simulink model "subsys"  (R2018a)
settings: Solver=VariableStepAuto  StartTime=0.0  StopTime=30  RelTol=1e-3
values from neighbouring files (symbols this model uses):
  p = polyfit(x,d,7)    [matlab.m]
undefined symbols (not defined in the file or in its folder): J, magnitude
libraries: simulink x9, visionstatistics x1, neural x1, dspsrcs4 x1, dspxfrm3 x1, dspsigops x1
settings Model: Creator=Thinkpad  LastModifiedBy=Administrator

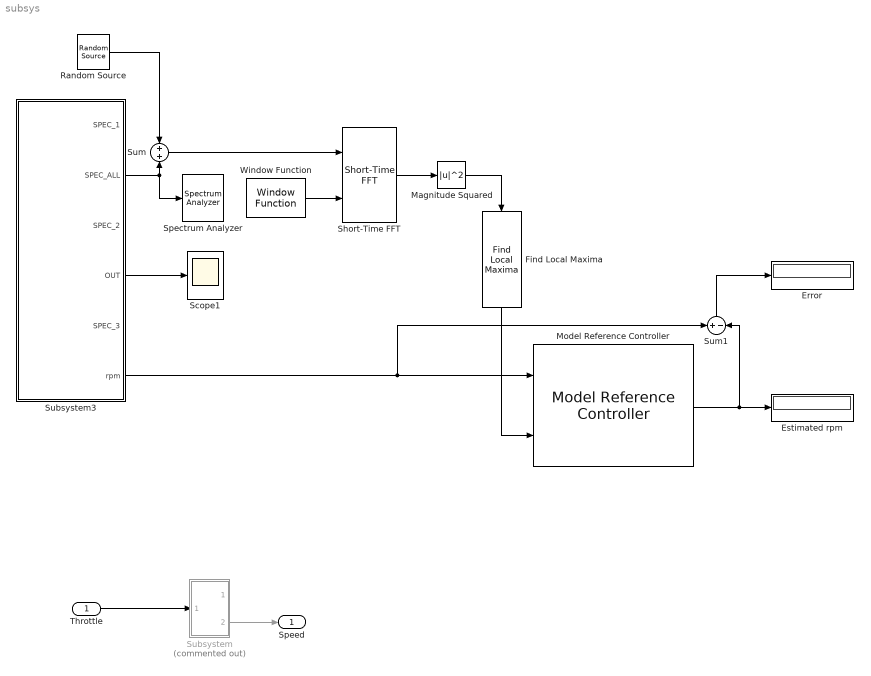
== system subsys ==
  Throttle : Inport
  Error : Display
  Estimated rpm : Display
  Find Local Maxima : visionstatistics/Find Local Maxima  num_peaks=2  nhood_size=[5 7]  src_thresh=Obsolete9b  src_thresh_inuse=Specify via dialog  threshold=10  inputIsHough=off  dt_peak=uint32  isOutVarDim=on  dt_count=uint32
      settings: SourceProductName=Computer Vision System Toolbox  SourceProductBaseCode=VP
  Magnitude Squared : Math  Operator=magnitude^2  SaturateOnIntegerOverflow=on
  Model Reference Controller : neural/Control Systems/Model Reference Controller  Nrc=[]  Nic=[]  Njc=[]  IW_y=[]  IW_u=[]  IW_r=[]  B1_c=[]  B2_c=[]  LW_c=[]  retraining_c=[]  max_i_int=[]  min_i_int=[]  max_r_int=[]  min_r_int=[]  Ts=[]  S1=[]  Ni=[]  Nj=[]  sim_file=0  trainfun=trainlm  Use_validation=[]  Use_Testing=[]  Use_Inc_training=[]  Use_previous_weights=[]  max_i=[]  min_i=[]  max_r=[]  min_r=[]  sam_training=[]  sam_training_c=[]  epochs=[]  epochs_c=[]  minp=[]  maxp=[]  mint=[]  maxt=[]  Normalize=[]  IW=[]  LW1_2=[]  LW2_1=[]  B1=[]  B2=[]  S1c=[]  Limit_output=[]  min_output=[]  max_output=[]  Ref_file=0
      settings: SourceProductName=Neural Network Toolbox  SourceProductBaseCode=NN
  Random Source : dspsrcs4/Random Source  SrcType=Gaussian  NormMethod=Ziggurat  CltLength=12  MinVal=0  MaxVal=1  MeanVal=0  VarVal=(0.05)^2  RepMode=Repeatable  rawSeed=1  IsInherit=off  SampMode=Discrete  SampTime=1/22050  SampFrame=512  DataType=Double  OutComplex=Real  OutputFrames=off
  Scope1 : Scope
  Short-Time FFT : dspxfrm3/Short-Time FFT  W=512  OvLap=384  M=1024
      settings: SourceProductName=DSP System Toolbox  SourceProductBaseCode=DS
  Spectrum Analyzer : SpectrumAnalyzer
  Subsystem : Subsystem  Commented=on
  Subsystem3 : Subsystem
  Sum : Sum
  Sum1 : Sum  Inputs=+-
  Window Function : dspsigops/Window Function  winmode=Generate window  wintype=Hamming  sampmode=Discrete  samptime=inf  N=512  Rs=50  beta=10  winsamp=Symmetric  UserWindow=hamming  OptParams=off  UserParams={'symmetric'}  dataType=double  isSigned=on  wordLen=16  udDataType=sfix(16)  fracBitsMode=Best precision  numFracBits=15  roundingMode=Floor  overflowMode=off  numSidelobes=4  sidelobeLevel=-30
      settings: SourceProductName=DSP System Toolbox  SourceProductBaseCode=DS
  Speed : Outport
  wires:
  Subsystem3/2(SPEC_ALL) -> Spectrum Analyzer/1, Sum/2
  Subsystem3/4(OUT) -> Scope1/1
  Window Function/1 -> Short-Time FFT/2
  Random Source/1 -> Sum/1
  Sum/1 -> Short-Time FFT/1
  Short-Time FFT/1 -> Magnitude Squared/1
  Magnitude Squared/1 -> Find Local Maxima/1
  Subsystem3/6(rpm) -> Sum1/1, Model Reference Controller/1
  Find Local Maxima/1 -> Model Reference Controller/2
  Model Reference Controller/1 -> Sum1/2, Estimated rpm/1
  Sum1/1 -> Error/1
  Throttle/1 -> Subsystem/1(Throttle)
  Subsystem/2(Speed) -> Speed/1

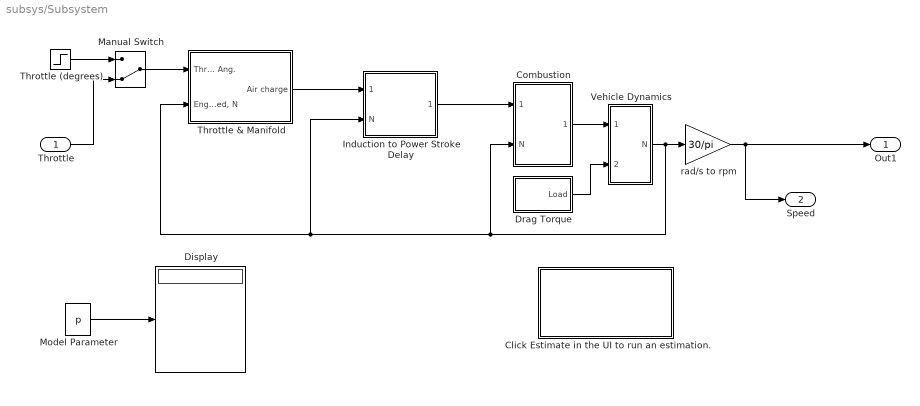
== system subsys/Subsystem ==
  Throttle : Inport
  Click Estimate in the UI to run an estimation. : Subsystem
      settings: OpenFcn=sdotool( slResolve('spe_speed_sdosession', 'spe_speed') );
      mask Display: disp('Parameter Estimation\nwith preloaded data')
  Combustion : Subsystem
  Display : Display
  Drag Torque : Subsystem
  Induction to Power Stroke Delay : Subsystem
  Manual Switch : ManualSwitch  CurrentSetting=0
  Model Parameter : Constant  Value=p
  Throttle (degrees) : Step  Time=2  Before=8.973  After=11  SampleTime=0
  Throttle & Manifold : Subsystem
  Vehicle Dynamics : Subsystem
  rad/s to rpm : Gain  Gain=30/pi  SaturateOnIntegerOverflow=on  OutDataTypeStr=Inherit: Same as input  ParamDataTypeStr=Inherit: Same as input
  Out1 : Outport
  Speed : Outport  Port=2
  wires:
  Model Parameter/1 -> Display/1
  Drag Torque/1(Load) -> Vehicle Dynamics/2(Tload)
  rad/s to rpm/1 -> Speed/1, Out1/1
  Throttle (degrees)/1 -> Manual Switch/1
  Throttle/1 -> Manual Switch/2
  Vehicle Dynamics/1(N) -> rad/s to rpm/1, Combustion/2(N), Throttle & Manifold/2("Engine Speed, N"), Induction to Power Stroke Delay/2(N)
  Manual Switch/1 -> Throttle & Manifold/1(Throttle Ang.)
  Induction to Power Stroke Delay/1(Air Charge) -> Combustion/1(Air Charge)
  Throttle & Manifold/1(Air charge) -> Induction to Power Stroke Delay/1(Air charge)
  Combustion/1(Torque) -> Vehicle Dynamics/1(Teng)

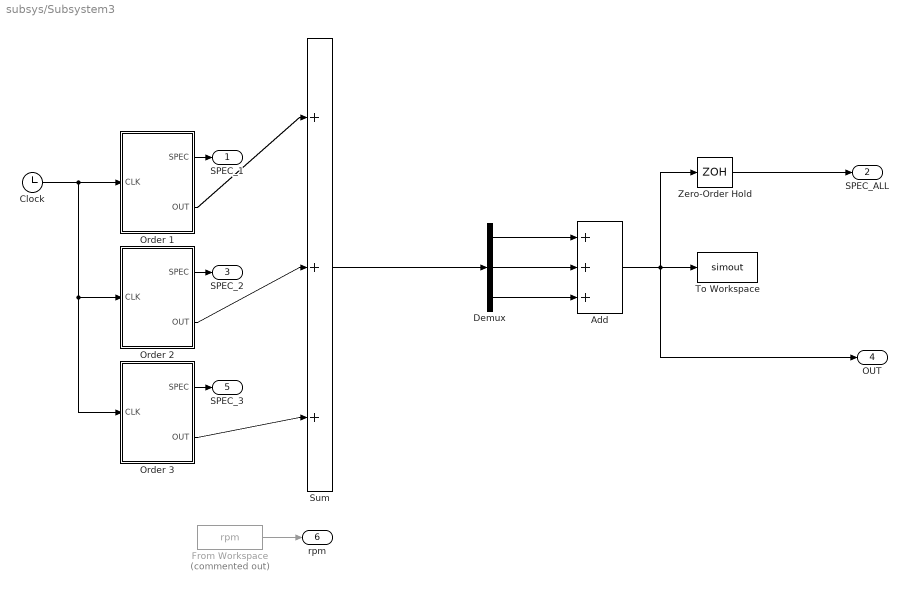
== system subsys/Subsystem3 ==
  Add : Sum  Inputs=+++
  Clock : Clock
  Demux : Demux  Outputs=3
  From Workspace : FromWorkspace  Commented=on  VariableName=rpm  SampleTime=0
  Order 1 : Subsystem
      mask DialogControl NVH_signal_generator Prompt: NVH signal generator
  Order 2 : Subsystem
      mask DialogControl NVH_signal_generator Prompt: NVH signal generator
  Order 3 : Subsystem
      mask DialogControl NVH_signal_generator Prompt: NVH signal generator
  Sum : Sum  Inputs=|+++
  To Workspace : ToWorkspace  VariableName=simout  SaveFormat=Structure With Time  SampleTime=-1
  Zero-Order Hold : ZeroOrderHold  SampleTime=-1
  SPEC_1 : Outport
  SPEC_ALL : Outport  Port=2
  SPEC_2 : Outport  Port=3
  OUT : Outport  Port=4
  SPEC_3 : Outport  Port=5
  rpm : Outport  Port=6
  wires:
  Clock/1 -> Order 3/1(CLK), Order 2/1(CLK), Order 1/1(CLK)
  Order 1/2(OUT) -> Sum/1
  Demux/1 -> Add/1
  Order 2/2(OUT) -> Sum/2
  Demux/2 -> Add/2
  Order 3/2(OUT) -> Sum/3
  Add/1 -> OUT/1, Zero-Order Hold/1, To Workspace/1
  Demux/3 -> Add/3
  Sum/1 -> Demux/1
  Order 3/1(SPEC) -> SPEC_3/1
  Zero-Order Hold/1 -> SPEC_ALL/1
  Order 2/1(SPEC) -> SPEC_2/1
  Order 1/1(SPEC) -> SPEC_1/1
  From Workspace/1 -> rpm/1

== system subsys/Subsystem/Click Estimate in the UI to run an estimation. ==

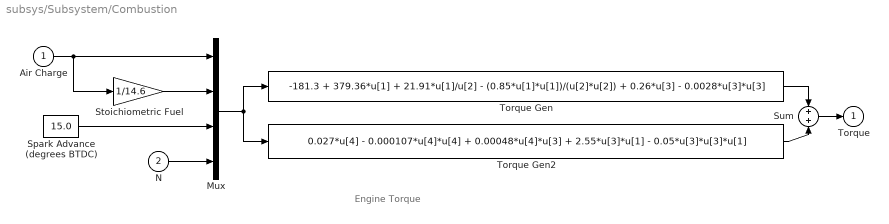
== system subsys/Subsystem/Combustion ==
  note: Engine Torque
  Air Charge : Inport
  N : Inport  Port=2
  Mux : Mux
  Spark Advance (degrees BTDC) : Constant  Value=15.0
  Stoichiometric Fuel : Gain  Gain=1/14.6  SaturateOnIntegerOverflow=on  OutDataTypeStr=Inherit: Same as input  ParamDataTypeStr=Inherit: Same as input
  Sum : Sum  SaturateOnIntegerOverflow=on  InputSameDT=on  OutDataTypeStr=Inherit: Same as first input
  Torque Gen : Fcn  Expr=-181.3 + 379.36*u[1] + 21.91*u[1]/u[2] - (0.85*u[1]*u[1])/(u[2]*u[2]) + 0.26*u[3] - 0.0028*u[3]*u[3]
  Torque Gen2 : Fcn  Expr=0.027*u[4] - 0.000107*u[4]*u[4] + 0.00048*u[4]*u[3] + 2.55*u[3]*u[1] - 0.05*u[3]*u[3]*u[1]
  Torque : Outport  InitialOutput=0
  wires:
  Stoichiometric Fuel/1 -> Mux/2
  Spark Advance (degrees BTDC)/1 -> Mux/3
  N/1 -> Mux/4
  Air Charge/1 -> Stoichiometric Fuel/1, Mux/1
  Mux/1 -> Torque Gen/1, Torque Gen2/1
  Torque Gen2/1 -> Sum/2
  Torque Gen/1 -> Sum/1
  Sum/1 -> Torque/1

== system subsys/Subsystem/Drag Torque ==
  note: Torque Disturbances
  Step : Step  Time=2  Before=25  After=25  SampleTime=0
  Step1 : Step  Time=8  After=0  SampleTime=0
  Sum1 : Sum  SaturateOnIntegerOverflow=on  InputSameDT=on  OutDataTypeStr=Inherit: Same as first input
  Load : Outport  InitialOutput=0
  wires:
  Step1/1 -> Sum1/2
  Step/1 -> Sum1/1
  Sum1/1 -> Load/1

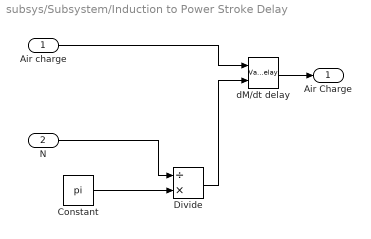
== system subsys/Subsystem/Induction to Power Stroke Delay ==
  Air charge : Inport
  N : Inport  Port=2
  Constant : Constant  Value=pi
  Divide : Product  Inputs=/*
  dM/dt delay : VariableTransportDelay  MaximumDelay=20  InitialOutput=0.152  MaximumPoints=3072  ZeroDelay=on  PadeOrder=2
  Air Charge : Outport
  wires:
  dM/dt delay/1 -> Air Charge/1
  Constant/1 -> Divide/2
  Divide/1 -> dM/dt delay/2
  Air charge/1 -> dM/dt delay/1
  N/1 -> Divide/1

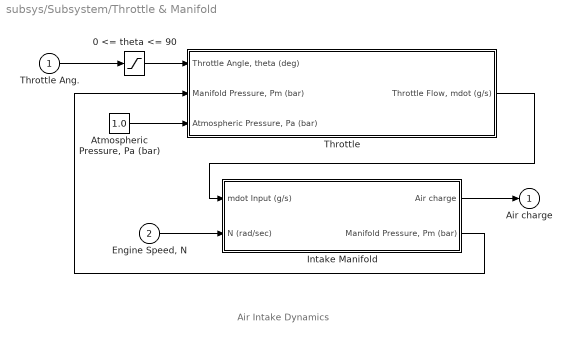
== system subsys/Subsystem/Throttle & Manifold ==
  note: Air Intake Dynamics
  Throttle Ang. : Inport
  "Engine Speed, N" : Inport  Port=2
  0 <= theta <= 90 : Saturate  UpperLimit=90  LowerLimit=0
  "Atmospheric Pressure, Pa (bar)" : Constant  Value=1.0
  Intake Manifold : Subsystem
  Throttle : Subsystem
  Air charge : Outport  InitialOutput=0
  wires:
  "Atmospheric Pressure, Pa (bar)"/1 -> Throttle/3("Atmospheric Pressure, Pa (bar) ")
  Intake Manifold/1(Air charge) -> Air charge/1
  Intake Manifold/2("Manifold Pressure, Pm (bar)") -> Throttle/2("Manifold Pressure, Pm (bar)")
  "Engine Speed, N"/1 -> Intake Manifold/2(N (rad/sec))
  Throttle/1("Throttle Flow, mdot (g/s)") -> Intake Manifold/1(mdot Input (g/s))
  Throttle Ang./1 -> 0 <= theta <= 90/1
  0 <= theta <= 90/1 -> Throttle/1("Throttle Angle, theta (deg)")

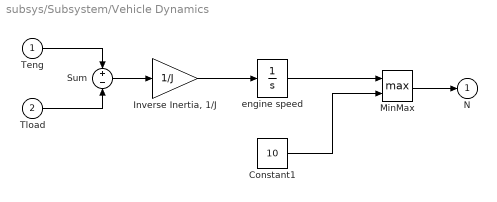
== system subsys/Subsystem/Vehicle Dynamics ==
  Teng : Inport
  Tload : Inport  Port=2
  Constant1 : Constant  Value=10
  "Inverse Inertia, 1/J" : Gain  Gain=1/J  SaturateOnIntegerOverflow=on  OutDataTypeStr=Inherit: Same as input  ParamDataTypeStr=Inherit: Same as input
  MinMax : MinMax  Function=max  Inputs=2
  Sum : Sum  Inputs=+-  SaturateOnIntegerOverflow=on  InputSameDT=on  OutDataTypeStr=Inherit: Same as first input
  engine speed : Integrator  InitialCondition=209.48
  N : Outport  InitialOutput=0
  wires:
  "Inverse Inertia, 1/J"/1 -> engine speed/1
  Sum/1 -> "Inverse Inertia, 1/J"/1
  Teng/1 -> Sum/1
  Tload/1 -> Sum/2
  MinMax/1 -> N/1
  engine speed/1 -> MinMax/1
  Constant1/1 -> MinMax/2

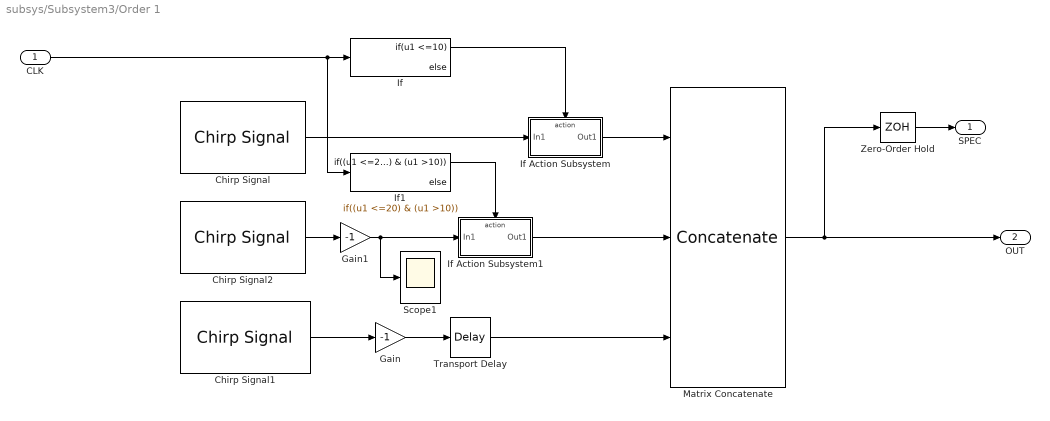
== system subsys/Subsystem3/Order 1 ==
  CLK : Inport
  Chirp Signal : simulink/Sources/Chirp Signal  f1=0.1  T=10  f2=1000
  Chirp Signal1 : simulink/Sources/Chirp Signal  f1=1000  T=10  f2=0.1
  Chirp Signal2 : simulink/Sources/Chirp Signal  f1=1000  T=10  f2=1000
  Gain : Gain  Gain=-1
  Gain1 : Gain  Gain=-1
  If : If  IfExpression=u1 <=10
  If Action Subsystem : Subsystem  TreatAsAtomicUnit=on
  If Action Subsystem1 : Subsystem  TreatAsAtomicUnit=on
  If1 : If  IfExpression=(u1 <=20) & (u1 >10)
  Matrix Concatenate : Concatenate  NumInputs=3
  Scope1 : Scope
  Transport Delay : TransportDelay  DelayTime=20
  Zero-Order Hold : ZeroOrderHold  SampleTime=-1
  SPEC : Outport
  OUT : Outport  Port=2
  wires:
  Gain1/1 -> Scope1/1, If Action Subsystem1/1(In1)
  CLK/1 -> If1/1, If/1
  Matrix Concatenate/1 -> OUT/1, Zero-Order Hold/1
  Gain/1 -> Transport Delay/1
  Transport Delay/1 -> Matrix Concatenate/3
  Chirp Signal2/1 -> Gain1/1
  If1/1 -> If Action Subsystem1/Action
  If/1 -> If Action Subsystem/Action
  Chirp Signal1/1 -> Gain/1
  If Action Subsystem/1(Out1) -> Matrix Concatenate/1
  If Action Subsystem1/1(Out1) -> Matrix Concatenate/2
  Chirp Signal/1 -> If Action Subsystem/1(In1)
  Zero-Order Hold/1 -> SPEC/1

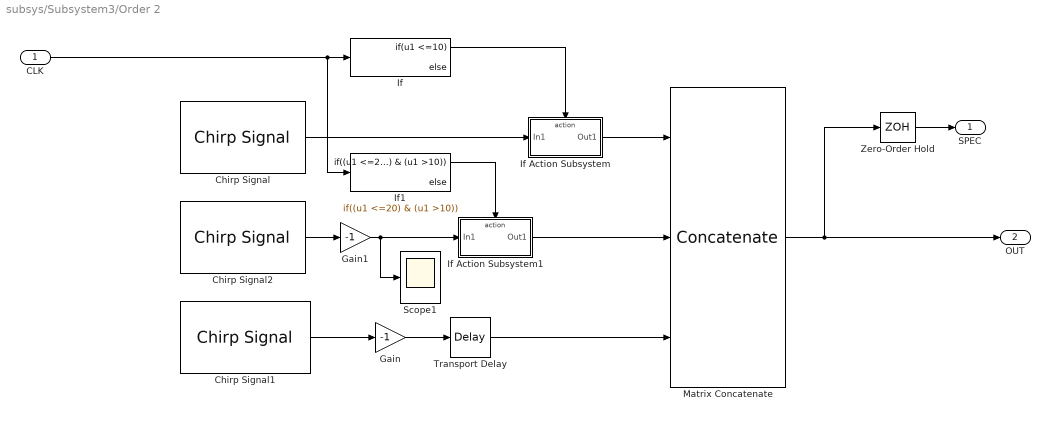
== system subsys/Subsystem3/Order 2 ==
  CLK : Inport
  Chirp Signal : simulink/Sources/Chirp Signal  f1=0.1  T=10  f2=4000
  Chirp Signal1 : simulink/Sources/Chirp Signal  f1=4000  T=10  f2=0.1
  Chirp Signal2 : simulink/Sources/Chirp Signal  f1=4000  T=10  f2=4000
  Gain : Gain  Gain=-1
  Gain1 : Gain  Gain=-1
  If : If  IfExpression=u1 <=10
  If Action Subsystem : Subsystem  TreatAsAtomicUnit=on
  If Action Subsystem1 : Subsystem  TreatAsAtomicUnit=on
  If1 : If  IfExpression=(u1 <=20) & (u1 >10)
  Matrix Concatenate : Concatenate  NumInputs=3
  Scope1 : Scope
  Transport Delay : TransportDelay  DelayTime=20
  Zero-Order Hold : ZeroOrderHold  SampleTime=-1
  SPEC : Outport
  OUT : Outport  Port=2
  wires:
  Gain1/1 -> Scope1/1, If Action Subsystem1/1(In1)
  CLK/1 -> If1/1, If/1
  Matrix Concatenate/1 -> OUT/1, Zero-Order Hold/1
  Gain/1 -> Transport Delay/1
  Transport Delay/1 -> Matrix Concatenate/3
  Chirp Signal2/1 -> Gain1/1
  If1/1 -> If Action Subsystem1/Action
  If/1 -> If Action Subsystem/Action
  Chirp Signal1/1 -> Gain/1
  If Action Subsystem/1(Out1) -> Matrix Concatenate/1
  If Action Subsystem1/1(Out1) -> Matrix Concatenate/2
  Chirp Signal/1 -> If Action Subsystem/1(In1)
  Zero-Order Hold/1 -> SPEC/1

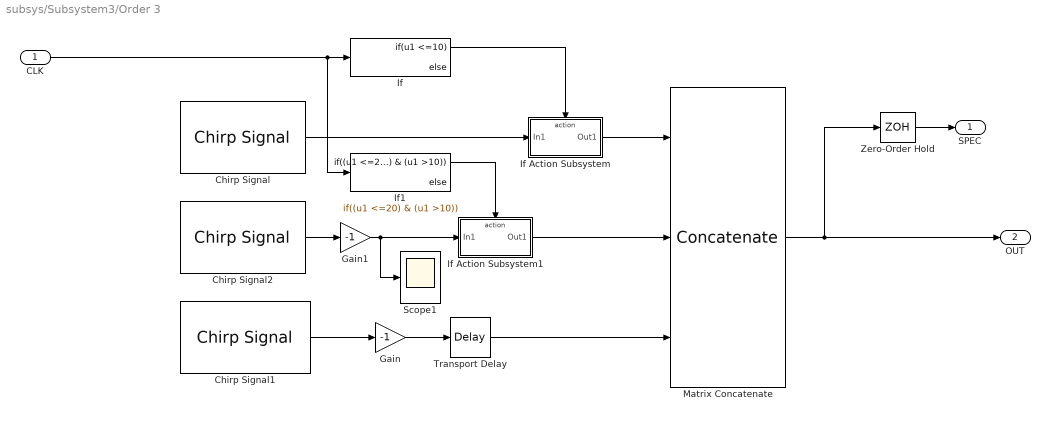
== system subsys/Subsystem3/Order 3 ==
  CLK : Inport
  Chirp Signal : simulink/Sources/Chirp Signal  f1=0.1  T=10  f2=8000
  Chirp Signal1 : simulink/Sources/Chirp Signal  f1=8000  T=10  f2=0.1
  Chirp Signal2 : simulink/Sources/Chirp Signal  f1=8000  T=10  f2=8000
  Gain : Gain  Gain=-1
  Gain1 : Gain  Gain=-1
  If : If  IfExpression=u1 <=10
  If Action Subsystem : Subsystem  TreatAsAtomicUnit=on
  If Action Subsystem1 : Subsystem  TreatAsAtomicUnit=on
  If1 : If  IfExpression=(u1 <=20) & (u1 >10)
  Matrix Concatenate : Concatenate  NumInputs=3
  Scope1 : Scope
  Transport Delay : TransportDelay  DelayTime=20
  Zero-Order Hold : ZeroOrderHold  SampleTime=-1
  SPEC : Outport
  OUT : Outport  Port=2
  wires:
  Gain1/1 -> Scope1/1, If Action Subsystem1/1(In1)
  CLK/1 -> If1/1, If/1
  Matrix Concatenate/1 -> OUT/1, Zero-Order Hold/1
  Gain/1 -> Transport Delay/1
  Transport Delay/1 -> Matrix Concatenate/3
  Chirp Signal2/1 -> Gain1/1
  If1/1 -> If Action Subsystem1/Action
  If/1 -> If Action Subsystem/Action
  Chirp Signal1/1 -> Gain/1
  If Action Subsystem/1(Out1) -> Matrix Concatenate/1
  If Action Subsystem1/1(Out1) -> Matrix Concatenate/2
  Chirp Signal/1 -> If Action Subsystem/1(In1)
  Zero-Order Hold/1 -> SPEC/1

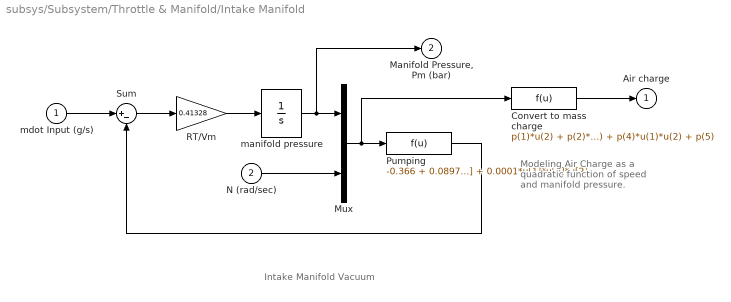
== system subsys/Subsystem/Throttle & Manifold/Intake Manifold ==
  note: Intake Manifold Vacuum
  note: Modeling Air Charge as a
      | quadratic function of speed
      | and manifold pressure.
  mdot Input (g/s) : Inport
  N (rad/sec) : Inport  Port=2
  Convert to mass charge : Fcn  Expr=p(1)*u(2) + p(2)*u(1) + p(3)*u(1)*u(1) + p(4)*u(1)*u(2) + p(5)
  Mux : Mux  Inputs=2
  Pumping : Fcn  Expr=-0.366 + 0.08979*u[1]*u[2] - 0.0337*u[2]*u[1]*u[1] + 0.0001*u[1]*u[2]*u[2]
  RT/Vm : Gain  Gain=0.41328  SaturateOnIntegerOverflow=on  OutDataTypeStr=Inherit: Same as input  ParamDataTypeStr=Inherit: Same as input
  Sum : Sum  Inputs=|+-  SaturateOnIntegerOverflow=on  InputSameDT=on  OutDataTypeStr=Inherit: Same as first input
  manifold pressure : Integrator  InitialCondition=0.543
  Air charge : Outport  InitialOutput=0
  "Manifold Pressure, Pm (bar)" : Outport  Port=2  InitialOutput=0
  wires:
  Pumping/1 -> Sum/2
  Sum/1 -> RT/Vm/1
  manifold pressure/1 -> "Manifold Pressure, Pm (bar)"/1, Mux/1
  Mux/1 -> Pumping/1, Convert to mass charge/1
  N (rad/sec)/1 -> Mux/2
  RT/Vm/1 -> manifold pressure/1
  mdot Input (g/s)/1 -> Sum/1
  Convert to mass charge/1 -> Air charge/1

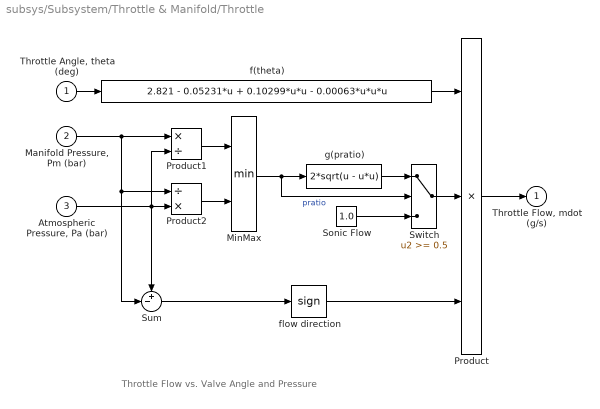
== system subsys/Subsystem/Throttle & Manifold/Throttle ==
  note: Throttle Flow vs. Valve Angle and Pressure
  "Throttle Angle, theta (deg)" : Inport
  "Manifold Pressure, Pm (bar)" : Inport  Port=2
  "Atmospheric Pressure, Pa (bar) " : Inport  Port=3
  MinMax : MinMax  Inputs=2  SaturateOnIntegerOverflow=on  InputSameDT=on
  Product : Product  Inputs=3  SaturateOnIntegerOverflow=on  RndMeth=Zero  InputSameDT=on  OutDataTypeStr=Inherit: Same as first input
  Product1 : Product  Inputs=*/  SaturateOnIntegerOverflow=on  RndMeth=Zero  InputSameDT=on  OutDataTypeStr=Inherit: Same as first input
  Product2 : Product  Inputs=/*  SaturateOnIntegerOverflow=on  RndMeth=Zero  InputSameDT=on  OutDataTypeStr=Inherit: Same as first input
  "Sonic Flow " : Constant  Value=1.0
  Sum : Sum  Inputs=+-|  SaturateOnIntegerOverflow=on  InputSameDT=on  OutDataTypeStr=Inherit: Same as first input
  Switch : Switch  Threshold=0.5  SaturateOnIntegerOverflow=on  InputSameDT=on
  f(theta) : Fcn  Expr=2.821 - 0.05231*u + 0.10299*u*u - 0.00063*u*u*u
  flow direction : Signum
  g(pratio) : Fcn  Expr=2*sqrt(u - u*u)
  "Throttle Flow, mdot (g/s)" : Outport  InitialOutput=0
  wires:
  f(theta)/1 -> Product/1
  Product/1 -> "Throttle Flow, mdot (g/s)"/1
  "Throttle Angle, theta (deg)"/1 -> f(theta)/1
  MinMax/1 -> g(pratio)/1, Switch/2  "pratio"
  Sum/1 -> flow direction/1
  flow direction/1 -> Product/3
  Switch/1 -> Product/2
  "Sonic Flow "/1 -> Switch/3
  g(pratio)/1 -> Switch/1
  "Atmospheric Pressure, Pa (bar) "/1 -> Product1/2, Product2/2, Sum/1
  Product1/1 -> MinMax/1
  Product2/1 -> MinMax/2
  "Manifold Pressure, Pm (bar)"/1 -> Product1/1, Product2/1, Sum/2

== system subsys/Subsystem3/Order 1/If Action Subsystem ==
  In1 : Inport
  Action Port : ActionPort  ActionType=then
  Out1 : Outport
  wires:
  In1/1 -> Out1/1

== system subsys/Subsystem3/Order 1/If Action Subsystem1 ==
  In1 : Inport
  Action Port : ActionPort  ActionType=then
  Out1 : Outport
  wires:
  In1/1 -> Out1/1

== system subsys/Subsystem3/Order 2/If Action Subsystem ==
  In1 : Inport
  Action Port : ActionPort  ActionType=then
  Out1 : Outport
  wires:
  In1/1 -> Out1/1

== system subsys/Subsystem3/Order 2/If Action Subsystem1 ==
  In1 : Inport
  Action Port : ActionPort  ActionType=then
  Out1 : Outport
  wires:
  In1/1 -> Out1/1

== system subsys/Subsystem3/Order 3/If Action Subsystem ==
  In1 : Inport
  Action Port : ActionPort  ActionType=then
  Out1 : Outport
  wires:
  In1/1 -> Out1/1

== system subsys/Subsystem3/Order 3/If Action Subsystem1 ==
  In1 : Inport
  Action Port : ActionPort  ActionType=then
  Out1 : Outport
  wires:
  In1/1 -> Out1/1
